simulink model "gm_AWFG_Phase2"  (R2018a)
settings: Solver=ode3  StartTime=0.0  StopTime=0.06  RelTol=1e-3  EnableMultiTasking=on
libraries: simulink x7, dspswit3 x1
Description:
  | AWFG_concept: This model explores the implementation concept
  | of an arbitrary waveform generator (AWFG) in a real-time target
  | platform with a combination of CPU and FPGA code.
  | This concepts aims at minimizing changes in the FPGA programming.
settings Model: Creator=Estra  LastModifiedBy=Talha Rao
settings SolverCC: PositivePriorityOrder=on
settings DataIOCC: LimitDataPoints=on  SaveFormat=Array
settings OptimizationCC: DefaultParameterBehavior=Inlined  UseDivisionForNetSlopeComputation=on  UseFloatMulNetSlope=on  InlineInvariantSignals=on  PassReuseOutputArgsAs=Individual arguments  ExpressionDepthLimit=2147483647  ZeroExternalMemoryAtStartup=off  ZeroInternalMemoryAtStartup=off  NoFixptDivByZeroProtection=on  EfficientFloat2IntCast=on  LifeSpan=1  MaxStackSize=64
settings DebuggingCC: SignalInfNanChecking=warning  UnderspecifiedInitializationDetection=Classic  MergeDetectMultiDrivingBlocksExec=none  SolverPrmCheckMsg=warning  ParameterTunabilityLossMsg=error  UniqueDataStoreMsg=warning  AllowSymbolicDim=off  StateNameClashWarn=warning  SFUnexpectedBacktrackingDiag=warning  SFNoUnconditionalDefaultTransitionDiag=warning  SFExecutionAtInitializationDiag=none
settings HardwareCC: ProdBitPerPointer=32  ProdBitPerSizeT=32  ProdBitPerPtrDiffT=32  ProdLargestAtomicInteger=Long  ProdLargestAtomicFloat=Double  ProdWordSize=32  ProdLongLongMode=on  ProdHWDeviceType=ARM Compatible->ARM Cortex  TargetBitPerPointer=64  TargetBitPerSizeT=64  TargetBitPerPtrDiffT=64  TargetLongLongMode=on  TargetIntDivRoundTo=Zero  TargetEndianess=LittleEndian  TargetWordSize=64  TargetHWDeviceType=Custom Processor->MATLAB Host Computer  ProdEqTarget=off
settings ModelReferenceCC: PropagateSignalLabelsOutOfModel=off
settings SFSimCC: MATLABDynamicMemAlloc=off
settings RTWCC: SystemTargetFile=ert.tlc  HardwareBoard=Xilinx Zynq-7000 based board  TLCOptions="-aInlineSetEventsForThisBaseRateFcn=TLC_FALSE -aSuppressMultiTaskScheduler=TLC_FALSE  -aRateBasedStepFcn=0"  TemplateMakefile=ert_default_tmf  GenerateReport=on  Toolchain=Xilinx Software Development Kit (SDK)  IncludeHyperlinkInReport=on  LaunchReport=on  GenerateTraceInfo=on  GenerateTraceReport=on  GenerateTraceReportSl=on  GenerateTraceReportSf=on  GenerateTraceReportEml=on  GenerateCodeMetricsReport=on
settings CodeAppCC: ForceParamTrailComments=on  IgnoreCustomStorageClasses=off  OperatorAnnotations=on  SimulinkDataObjDesc=on  SFDataObjDesc=on  CustomSymbolStrGlobalVar=rt$N$M  CustomSymbolStrType=$N$M  CustomSymbolStrFcn=$N$M$F  CustomSymbolStrMacro=$N$M  InsertBlockDesc=on
settings ERTTargetCC: IncludeMdlTerminateFcn=off  CombineSignalStateStructs=on  SupportAbsoluteTime=off  SupportComplex=off  SupportNonInlinedSFcns=on  SupportVariableSizeSignals=on  InlinedParameterPlacement=NonHierarchical  ERTFilePackagingFormat=CompactWithDataFile
settings ConfigComp: CovMetricSettings=dw  CovHtmlReporting=on  CovSaveCumulativeToWorkspaceVar=on  CovSaveSingleToWorkspaceVar=on  CovExternalEMLEnable=off

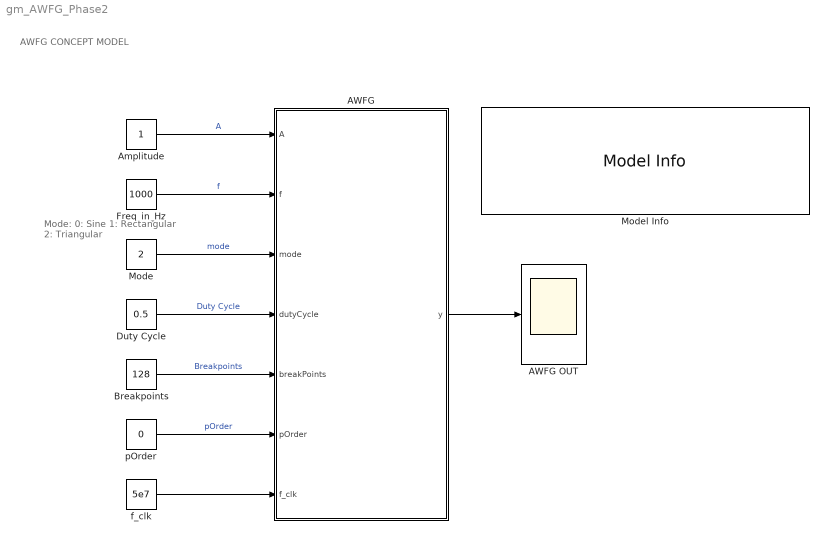
== system gm_AWFG_Phase2 ==
  note: AWFG CONCEPT MODEL
  note: Mode:
      | 0: Sine
      | 1: Rectangular
      | 2: Triangular
  AWFG : Subsystem
  AWFG OUT : Scope
  Amplitude : Constant  OutDataTypeStr=single
  Breakpoints : Constant  Value=128  OutDataTypeStr=single
  Duty Cycle : Constant  Value=0.5  OutDataTypeStr=single
  Freq_in_Hz : Constant  Value=1000  OutDataTypeStr=single
  Mode : Constant  Value=2  OutDataTypeStr=single
  Model Info : simulink/Model-Wide Utilities/Model Info  Frame=on  DisplayStringWithTags=|  HorizontalTextAlignment=Left  LeftAlignmentValue=0.02
      | Model Info
      | Creator:       R. Estrada, FH JOANNEUM, 2018
      | Modified by: %<ModifiedBy>
      | Modify Date: %<ModifiedDate>
      | Version:%<ModelVersion>
      | Description:
      | %<Description>
  f_clk : Constant  Value=5e7
  pOrder : Constant  Value=0  OutDataTypeStr=single
  wires:
  AWFG/1(y) -> AWFG OUT/1
  Amplitude/1 -> AWFG/1(A)  "A"
  Freq_in_Hz/1 -> AWFG/2(f)  "f"
  Mode/1 -> AWFG/3(mode)  "mode"
  Duty Cycle/1 -> AWFG/4(dutyCycle)  "Duty Cycle"
  Breakpoints/1 -> AWFG/5(breakPoints)  "Breakpoints"
  pOrder/1 -> AWFG/6(pOrder)  "pOrder"
  f_clk/1 -> AWFG/7(f_clk)

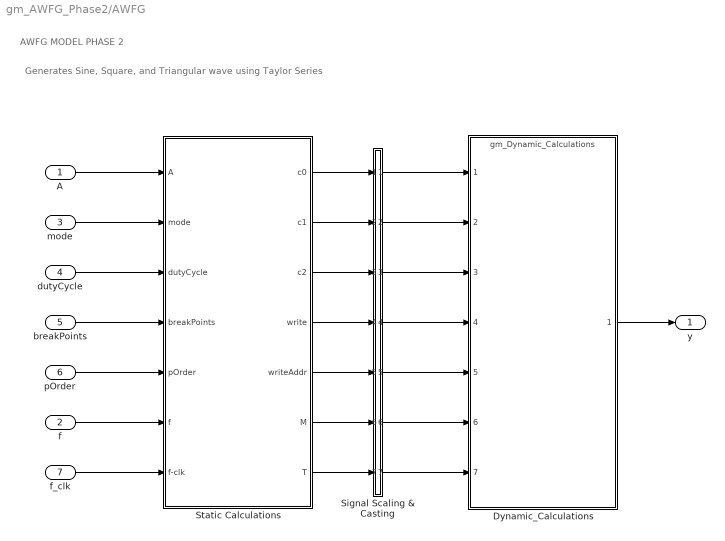
== system gm_AWFG_Phase2/AWFG ==
  note: Generates Sine, Square, and Triangular wave using Taylor Series
  note: AWFG MODEL PHASE 2
  A : Inport
  f : Inport  Port=2
  mode : Inport  Port=3
  dutyCycle : Inport  Port=4
  breakPoints : Inport  Port=5
  pOrder : Inport  Port=6
  f_clk : Inport  Port=7
  Dynamic_Calculations : ModelReference  ModelNameDialog=gm_Dynamic_Calculations  SimulationMode=Normal  Variant=on  OverrideUsingVariant=HDLC_internal_variant_GeneratedDUT  ModelReferenceVersion=1.506
  Signal Scaling & Casting : Subsystem
  Static Calculations : Subsystem
  y : Outport
  wires:
  Dynamic_Calculations/1 -> y/1
  A/1 -> Static Calculations/1(A)
  mode/1 -> Static Calculations/2(mode)
  dutyCycle/1 -> Static Calculations/3(dutyCycle)
  breakPoints/1 -> Static Calculations/4(breakPoints)
  pOrder/1 -> Static Calculations/5(pOrder)
  f/1 -> Static Calculations/6(f)
  f_clk/1 -> Static Calculations/7(f-clk)
  Signal Scaling & Casting/1(c0i) -> Dynamic_Calculations/1
  Signal Scaling & Casting/2(c1i) -> Dynamic_Calculations/2
  Signal Scaling & Casting/3(c2i) -> Dynamic_Calculations/3
  Signal Scaling & Casting/4(writei) -> Dynamic_Calculations/4
  Signal Scaling & Casting/5(writeAddri) -> Dynamic_Calculations/5
  Signal Scaling & Casting/6(Mi) -> Dynamic_Calculations/6
  Signal Scaling & Casting/7(Ti) -> Dynamic_Calculations/7
  Static Calculations/7(T) -> Signal Scaling & Casting/7(T)
  Static Calculations/6(M) -> Signal Scaling & Casting/6(M)
  Static Calculations/5(writeAddr) -> Signal Scaling & Casting/5(writeAddr)
  Static Calculations/4(write) -> Signal Scaling & Casting/4(write)
  Static Calculations/3(c2) -> Signal Scaling & Casting/3(c2)
  Static Calculations/2(c1) -> Signal Scaling & Casting/2(c1)
  Static Calculations/1(c0) -> Signal Scaling & Casting/1(c0)

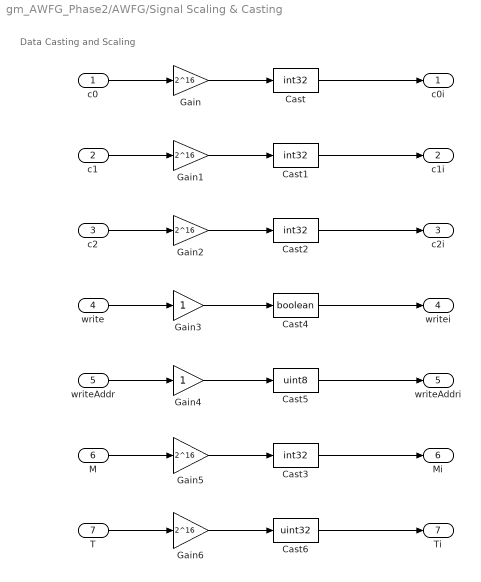
== system gm_AWFG_Phase2/AWFG/Signal Scaling & Casting ==
  note: Data Casting and Scaling
  c0 : Inport
  c1 : Inport  Port=2
  c2 : Inport  Port=3
  write : Inport  Port=4
  writeAddr : Inport  Port=5
  M : Inport  Port=6
  T : Inport  Port=7
  Cast{,1..3} (4 alike) : DataTypeConversion  OutDataTypeStr=int32
  Cast4 : DataTypeConversion  OutDataTypeStr=boolean
  Cast5 : DataTypeConversion  OutDataTypeStr=uint8
  Cast6 : DataTypeConversion  OutDataTypeStr=uint32
  Gain{,1..2,5..6} (5 alike) : Gain  Gain=2^16
  Gain3 : Gain
  Gain4 : Gain
  c0i : Outport
  c1i : Outport  Port=2
  c2i : Outport  Port=3
  writei : Outport  Port=4
  writeAddri : Outport  Port=5
  Mi : Outport  Port=6
  Ti : Outport  Port=7
  wires:
  c0/1 -> Gain/1
  c1/1 -> Gain1/1
  c2/1 -> Gain2/1
  write/1 -> Gain3/1
  writeAddr/1 -> Gain4/1
  M/1 -> Gain5/1
  T/1 -> Gain6/1
  Gain/1 -> Cast/1
  Gain1/1 -> Cast1/1
  Gain2/1 -> Cast2/1
  Gain3/1 -> Cast4/1
  Gain4/1 -> Cast5/1
  Gain5/1 -> Cast3/1
  Gain6/1 -> Cast6/1
  Cast6/1 -> Ti/1
  Cast3/1 -> Mi/1
  Cast5/1 -> writeAddri/1
  Cast4/1 -> writei/1
  Cast2/1 -> c2i/1
  Cast1/1 -> c1i/1
  Cast/1 -> c0i/1

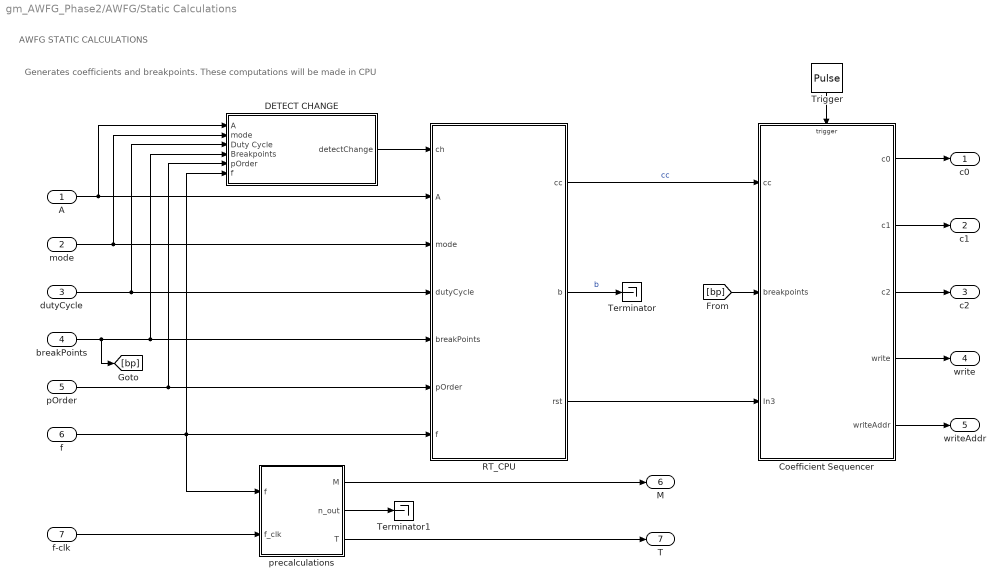
== system gm_AWFG_Phase2/AWFG/Static Calculations ==
  note: AWFG STATIC CALCULATIONS
  note: Generates coefficients and breakpoints. These computations will be made in CPU
  A : Inport
  mode : Inport  Port=2
  dutyCycle : Inport  Port=3
  breakPoints : Inport  Port=4
  pOrder : Inport  Port=5
  f : Inport  Port=6
  f-clk : Inport  Port=7
  Coefficient Sequencer : Subsystem
  DETECT CHANGE : Subsystem
  RT_CPU : MATLAB Function  TreatAsAtomicUnit=on
  Terminator : Terminator
  Terminator1 : Terminator
  Trigger : DiscretePulseGenerator  PulseType=Time based  Period=1/5e7  PulseWidth=50
  precalculations : Subsystem
  c0 : Outport
  c1 : Outport  Port=2
  c2 : Outport  Port=3
  write : Outport  Port=4
  writeAddr : Outport  Port=5
  M : Outport  Port=6
  T : Outport  Port=7
  wires:
  RT_CPU/1(cc) -> Coefficient Sequencer/1(cc)  "cc"
  f/1 -> precalculations/1(f), RT_CPU/7(f), DETECT CHANGE/6(f)
  breakPoints/1 -> [bp], DETECT CHANGE/4(Breakpoints), RT_CPU/5(breakPoints)
  f-clk/1 -> precalculations/2(f_clk)
  A/1 -> DETECT CHANGE/1(A), RT_CPU/2(A)
  pOrder/1 -> DETECT CHANGE/5(pOrder), RT_CPU/6(pOrder)
  precalculations/2(n_out) -> Terminator1/1
  mode/1 -> RT_CPU/3(mode), DETECT CHANGE/2(mode)
  dutyCycle/1 -> DETECT CHANGE/3(Duty Cycle), RT_CPU/4(dutyCycle)
  DETECT CHANGE/1(detectChange) -> RT_CPU/1(ch)
  precalculations/3(T) -> T/1
  precalculations/1(M) -> M/1
  Trigger/1 -> Coefficient Sequencer/Trigger
  RT_CPU/3(rst) -> Coefficient Sequencer/3(In3)
  [bp] -> Coefficient Sequencer/2(breakpoints)
  Coefficient Sequencer/1(c0) -> c0/1
  Coefficient Sequencer/2(c1) -> c1/1
  Coefficient Sequencer/3(c2) -> c2/1
  Coefficient Sequencer/4(write) -> write/1
  Coefficient Sequencer/5(writeAddr) -> writeAddr/1
  RT_CPU/2(b) -> Terminator/1  "b"

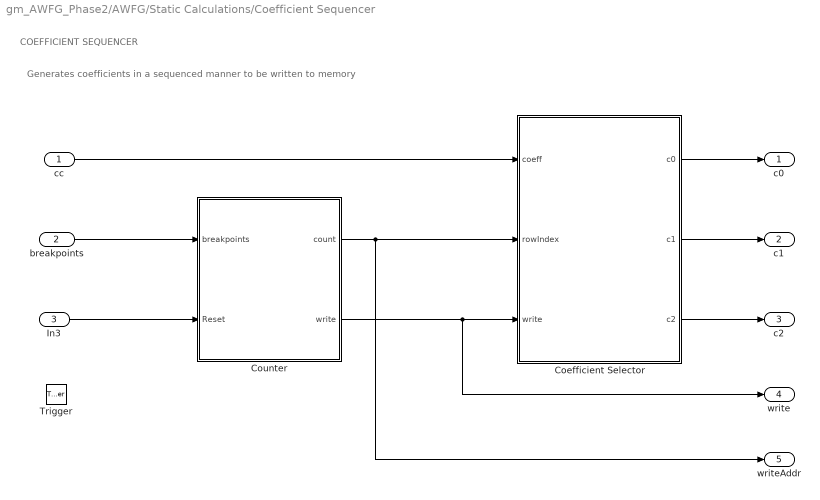
== system gm_AWFG_Phase2/AWFG/Static Calculations/Coefficient Sequencer ==
  note: COEFFICIENT SEQUENCER
  note: Generates coefficients in a sequenced manner to be written to memory
  cc : Inport
  breakpoints : Inport  Port=2
  In3 : Inport  Port=3
  Trigger : TriggerPort  VariantControl=Variant  PortDimensions=1
  Coefficient Selector : Subsystem
  Counter : Subsystem
  c0 : Outport
  c1 : Outport  Port=2
  c2 : Outport  Port=3
  write : Outport  Port=4
  writeAddr : Outport  Port=5
  wires:
  breakpoints/1 -> Counter/1(breakpoints)
  In3/1 -> Counter/2(Reset)
  cc/1 -> Coefficient Selector/1(coeff)
  Counter/1(count) -> writeAddr/1, Coefficient Selector/2(rowIndex)
  Counter/2(write) -> write/1, Coefficient Selector/3(write)
  Coefficient Selector/1(c0) -> c0/1
  Coefficient Selector/2(c1) -> c1/1
  Coefficient Selector/3(c2) -> c2/1

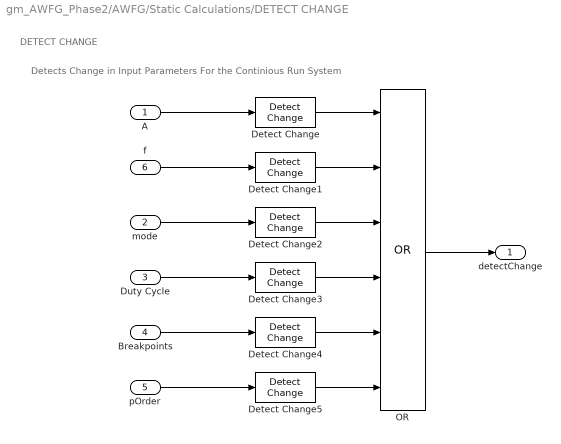
== system gm_AWFG_Phase2/AWFG/Static Calculations/DETECT CHANGE ==
  note: Detects Change in Input Parameters For the Continious Run System
  note: DETECT CHANGE
  A : Inport
  mode : Inport  Port=2
  Duty Cycle : Inport  Port=3
  Breakpoints : Inport  Port=4
  pOrder : Inport  Port=5
  f : Inport  Port=6
  Detect Change{,1..5} (6 alike) : simulink/Logic and Bit Operations/Detect Change  vinit=0  OutDataTypeStr=boolean
  OR : Logic  Operator=OR  Inputs=6  AllPortsSameDT=off  OutDataTypeStr=boolean
  detectChange : Outport
  wires:
  Detect Change3/1 -> OR/4
  mode/1 -> Detect Change2/1
  Detect Change5/1 -> OR/6
  Detect Change1/1 -> OR/2
  Breakpoints/1 -> Detect Change4/1
  pOrder/1 -> Detect Change5/1
  Detect Change4/1 -> OR/5
  Detect Change2/1 -> OR/3
  Detect Change/1 -> OR/1
  Duty Cycle/1 -> Detect Change3/1
  f/1 -> Detect Change1/1
  A/1 -> Detect Change/1
  OR/1 -> detectChange/1

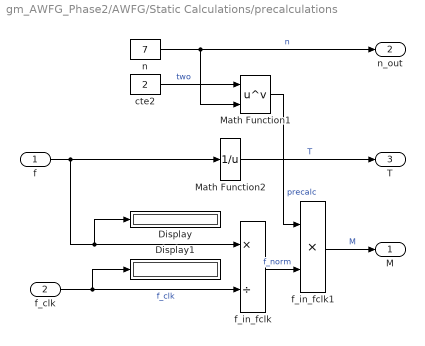
== system gm_AWFG_Phase2/AWFG/Static Calculations/precalculations ==
  f : Inport
  f_clk : Inport  Port=2
  Display : Display
  Display1 : Display
  Math Function1 : Math  Operator=pow  SaturateOnIntegerOverflow=on
  Math Function2 : Math  Operator=reciprocal  SaturateOnIntegerOverflow=on
  cte2 : Constant  Value=2  SampleTime=-1
  f_in_fclk : Product  Inputs=*/
  f_in_fclk1 : Product  Inputs=**
  n : Constant  Value=7  SampleTime=-1
  M : Outport
  n_out : Outport  Port=2
  T : Outport  Port=3
  wires:
  cte2/1 -> Math Function1/1  "two"
  n/1 -> Math Function1/2, n_out/1  "n"
  Math Function1/1 -> f_in_fclk1/1  "precalc"
  Math Function2/1 -> T/1  "T"
  f_in_fclk1/1 -> M/1  "M"
  f_clk/1 -> f_in_fclk/2, Display1/1  "f_clk"
  f_in_fclk/1 -> f_in_fclk1/2  "f_norm"
  f/1 -> Math Function2/1, Display/1, f_in_fclk/1

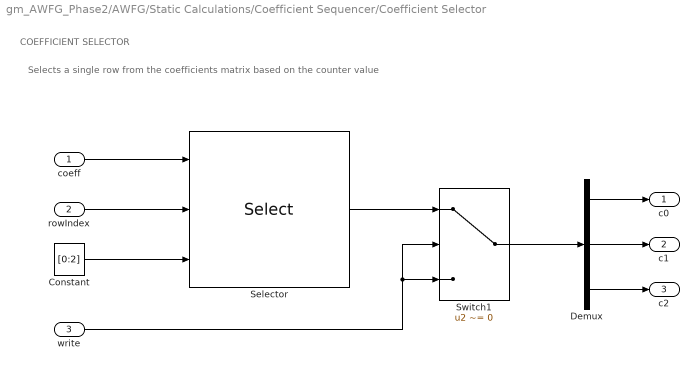
== system gm_AWFG_Phase2/AWFG/Static Calculations/Coefficient Sequencer/Coefficient Selector ==
  note: COEFFICIENT SELECTOR
  note: Selects a single row from the coefficients matrix based on the counter value
  coeff : Inport
  rowIndex : Inport  Port=2
  write : Inport  Port=3
  Constant : Constant  Value=[0:2]
  Demux : Demux  Outputs=3
  Selector : Selector  NumberOfDimensions=2  IndexMode=Zero-based  InputPortWidth=3  IndexOptions=Starting index (port),Index vector (port)  Indices=[1 3],[0 : 2]  OutputSizes=1,1
  Switch1 : Switch  Criteria=u2 ~= 0
  c0 : Outport
  c1 : Outport  Port=2
  c2 : Outport  Port=3
  wires:
  rowIndex/1 -> Selector/2
  coeff/1 -> Selector/1
  Selector/1 -> Switch1/1
  Demux/3 -> c2/1
  write/1 -> Switch1/2, Switch1/3
  Demux/2 -> c1/1
  Demux/1 -> c0/1
  Constant/1 -> Selector/3
  Switch1/1 -> Demux/1

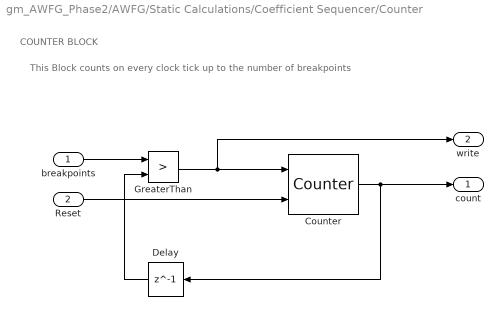
== system gm_AWFG_Phase2/AWFG/Static Calculations/Coefficient Sequencer/Counter ==
  note: This Block counts on every clock tick up to the number of breakpoints
  note: COUNTER BLOCK
  breakpoints : Inport
  Reset : Inport  Port=2
  Counter : dspswit3/Counter  Direction=Up  CountEvent=Non-zero sample  CounterSize=User defined  MaxCount=255  InitialCount=0  Output=Count  HitValue=32  ResetInput=on  SamplesPerFrame=1  Ts=1  CntDtype=single  HitDtype=Logical
  Delay : Delay  DelayLength=1
  GreaterThan : RelationalOperator  Operator=>  OutDataTypeStr=boolean  RndMeth=Simplest
  count : Outport
  write : Outport  Port=2
  wires:
  GreaterThan/1 -> write/1, Counter/1
  Counter/1 -> count/1, Delay/1
  breakpoints/1 -> GreaterThan/1
  Delay/1 -> GreaterThan/2
  Reset/1 -> Counter/2

== matlab function gm_AWFG_Phase2/AWFG/Static Calculations/RT_CPU ==
  data: ch input; A input [0..1]; mode input [0..2]; dutyCycle input [0..1]; breakPoints input [4..255]; pOrder input [0..3]; f input [0..10000]; cc output size=[256 4]; b output size=[1 255] [4..255]; rst output
function [cc,b,rst]  = fcn(ch,A,mode,dutyCycle, breakPoints,pOrder, f)
%% RT CPU
%   This Embedded Matlab function calculates the polynomial coefficients
%       and breaks points according to the external user settings. 
%       Three different waveforms can be selected with "mode"
%               0: Sine
%               1: Rectangular (not implemented yet)
%               2: Triangular  (not implemented yet)
%       
%    Author: R. Estrada, FH JOANNEUM, 2018
%
%%
    % Declaration of global variables
    persistent cc0 b0 i0;
    rst = single(0);
    if isempty(cc0)    
        cc0 = single(zeros(101,3));
        b0  = single(zeros(1,101));
        i0  = single(0);  %Used to checks if the program is running for the 1st time
    end
    
    
    if (ch || i0<1)        
        
        rst = single(1);
        i0=single(1);
        ch = 0;
        
        %Bound values of breakpoints
        assert(breakPoints<=256);
        
        cc = single(zeros(breakPoints+1,3));        %% Creates coefficients array 
        b  = single(zeros(1,(breakPoints + 1)));    %% Create breakpoints array 
        tf = single(1/f);
        y  = single(zeros(1 , (breakPoints + 1)));
        x= single(linspace(0,1,breakPoints+1));
        x1= single(linspace(0,1,breakPoints));
        
        switch mode
            case 0 % Sine wave
                                
                y  = A*sin(2*pi.*x);   
            
            case 1 % Square Wave  
                
                y = (x < dutyCycle).*(A) + (x >= dutyCycle).*(-A);
                y(breakPoints+1) = A;
                    
            case 2 % Triangular wave                
                
                if (dutyCycle ==0 || dutyCycle == 1)     %To avoid division by 0
                    
                    y = (dutyCycle == 1).*(-A+(x1*A*2)) +...
                        (dutyCycle ==0).*(-A+((1-x1)*A*2));
                    y= [y y(1)];
                else
                    
                    y = (x <= dutyCycle).*(-A+(x*A*(2/dutyCycle)))+...
                        (x > dutyCycle).*(-A+((1-x)*A*(2/(1-dutyCycle))));

                end
               
            otherwise
                y  = single(0);
        end

        %% Finite difference
        %   Coefficients
        cfd = [  1 0 0 0;...
                -1 1 0 0; ...
                 1 -2 1 0; ...
                -1 3 -3 1];

        % Extend array around the end
        yy = [y y(2:4)];
        
        for j=0:1:breakPoints                        % Sweep of break points
            b(1,j+1)=j*tf/breakPoints;               % Store actual break point
            ys = [yy(j+1) yy(j+2) yy(j+3) yy(j+4)];   % Prepare y vector
            for i=0:1:pOrder       
                dy = cfd(i+1,:) * ys'/(tf/breakPoints)^i; % Compute pOrder derivate        
                cc(j+1,i+1)= dy/factorial(i);        
            end                  
        end
        
        % Store values in global variables
        cc0 = cc;  
        b0  = b;
    else
        % Keep the previous values
        cc = cc0;
        b  = b0;
    end %end of main if
    
end % Function
